simulink model "C4"  (R2024a)
settings: Solver=VariableStepAuto  StartTime=0.0  StopTime=10.0  RelTol=1e-3

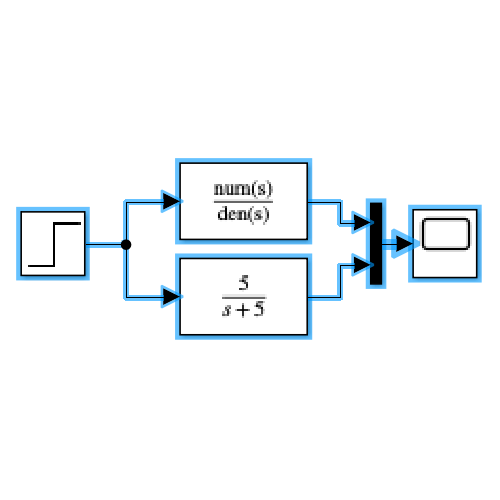
[thumbnail: Simulink's stored preview of the top-level diagram]
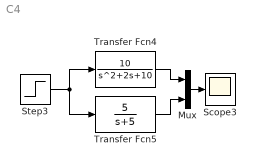
== system C4 ==
  Mux : Mux  Inputs=2
  Scope3 : Scope
  Step3 : Step  Time=0  After=2  SampleTime=0
  Transfer Fcn4 : TransferFcn  Numerator=[10]  Denominator=[1 2 10]
  Transfer Fcn5 : TransferFcn  Numerator=[5]  Denominator=[1 5]
  wires:
  Transfer Fcn4/1 -> Mux/1
  Transfer Fcn5/1 -> Mux/2
  Step3/1 -> Transfer Fcn5/1, Transfer Fcn4/1
  Mux/1 -> Scope3/1
